simulink model "offlineProcessing"  (R2014a)
settings: Solver=ode45  StartTime=0.0  StopTime=36  RelTol=1e-3
undefined symbols (not defined in the file or in its folder): FS, numSamplesPer20msFrame
libraries: dspxfrm3 x2, dspsigops x2, dspsrcs4 x1, dspsnks4 x1
settings Model: Creator=Abhi  LastModifiedBy=Abhi
settings DebuggingCC: SolverPrmCheckMsg=none

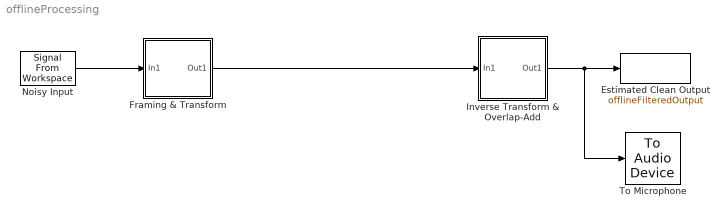
== system offlineProcessing ==
  Estimated Clean Output : ToWorkspace  VariableName=offlineFilteredOutput  SaveFormat=Structure  SampleTime=-1
      settings: Save2DSignal=2-D array (concatenate along first dimension)
  Framing & Transform : Subsystem
  Inverse Transform & Overlap-Add : Subsystem
  Noisy Input : dspsrcs4/Signal From Workspace  X=noisyInput  Ts=1/FS  nsamps=numSamplesPer20msFrame  OutputAfterFinalValue=Setting to zero  ignoreOrWarnInputAndFrameLengths=off
  To Microphone : dspsnks4/To Audio Device  deviceName=Default  inheritSampleRate=on  sampleRate=44100  deviceDatatype=Determine from input data type  autoBufferSize=on  bufferSize=4096  queueDuration=1.0  defaultOutputChannelMapping=on  outputChannelMapping=1:2
  wires:
  Noisy Input/1 -> Framing & Transform/1(In1)
  Inverse Transform & Overlap-Add/1(Out1) -> To Microphone/1, Estimated Clean Output/1
  Framing & Transform/1(Out1) -> Inverse Transform & Overlap-Add/1(In1)

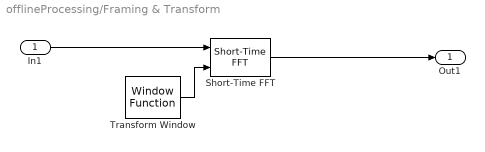
== system offlineProcessing/Framing & Transform ==
  In1 : Inport
  Short-Time FFT : dspxfrm3/Short-Time FFT  W=numSamplesPer20msFrame  OvLap=overlapSamples  M=numSamplesPer20msFrame  TreatMby1Signals=One channel
  Transform Window : dspsigops/Window Function  winmode=Generate window  wintype=Hanning  sampmode=Discrete  samptime=1  N=numSamplesPer20msFrame  Rs=50  beta=10  winsamp=Symmetric  UserWindow=hamming  OptParams=off  UserParams={'symmetric'}  RowConvenienceOn=on  dataType=double  isSigned=on  wordLen=16  udDataType=sfix(16)  fracBitsMode=Best precision  numFracBits=15  roundingMode=Floor  overflowMode=off  numSidelobes=4  sidelobeLevel=-30
  Out1 : Outport
  wires:
  Short-Time FFT/1 -> Out1/1
  Transform Window/1 -> Short-Time FFT/2
  In1/1 -> Short-Time FFT/1

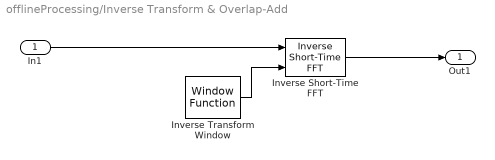
== system offlineProcessing/Inverse Transform & Overlap-Add ==
  In1 : Inport
  Inverse Transform Window : dspsigops/Window Function  winmode=Generate window  wintype=Hanning  sampmode=Discrete  samptime=1  N=numSamplesPer20msFrame  Rs=50  beta=10  winsamp=Symmetric  UserWindow=hamming  OptParams=off  UserParams={'symmetric'}  RowConvenienceOn=on  dataType=double  isSigned=on  wordLen=16  udDataType=sfix(16)  fracBitsMode=Best precision  numFracBits=15  roundingMode=Floor  overflowMode=off  numSidelobes=4  sidelobeLevel=-30
  Inverse Short-Time FFT : dspxfrm3/Inverse  Short-Time FFT  W=numSamplesPer20msFrame  OvLap=overlapSamples  OutFrameSize=numSamplesPer20msFrame  InConjSymm=on  DoAssert=off  Tol=1e-4
  Out1 : Outport
  wires:
  Inverse Short-Time FFT/1 -> Out1/1
  Inverse Transform Window/1 -> Inverse Short-Time FFT/2
  In1/1 -> Inverse Short-Time FFT/1
